simulink model "fig1"  (R2019b)
settings: Solver=VariableStepAuto  StartTime=0.0  StopTime=0.035  RelTol=1e-3
values from neighbouring files (symbols this model uses):
  f = 50    [Circuit_1.m]    (also in Circuit_2.m; Circuit_3_connected.m; Circuit_3_disconnected.m)
  V = (400*sqrt(2))/sqrt(3)    [Circuit_1.m]    (also in Circuit_2.m; Circuit_3_connected.m = (70*sqrt(2))/sqrt(3); Circuit_3_disconnected.m = (70*sqrt(2))/sqrt(3))
libraries: powerlib x8
settings Model: Creator=100448597  LastModifiedBy=robom
settings DataIOCC: SaveOutput=off  ReturnWorkspaceOutputs=off
settings SFSimCC: CustomCodeUndefinedFunction=UseInterfaceOnly

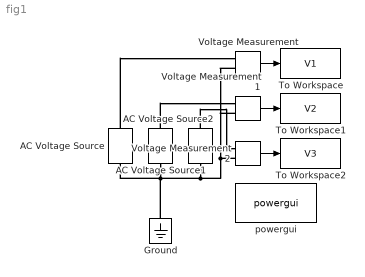
== system fig1 ==
  AC Voltage Source : powerlib/Electrical Sources/AC Voltage Source  Amplitude=V  Phase=0  Frequency=f  SampleTime=0  Measurements=None  BusType=swing  Pref=10e3  Qref=0  Qmin=-inf  Qmax=+inf
      settings: SourceProductName=Simscape Electrical
  AC Voltage Source1 : powerlib/Electrical Sources/AC Voltage Source  Amplitude=V  Phase=-120  Frequency=f  SampleTime=0  Measurements=None  BusType=swing  Pref=10e3  Qref=0  Qmin=-inf  Qmax=+inf
      settings: SourceProductName=Simscape Electrical
  AC Voltage Source2 : powerlib/Electrical Sources/AC Voltage Source  Amplitude=V  Phase=-240  Frequency=f  SampleTime=0  Measurements=None  BusType=swing  Pref=10e3  Qref=0  Qmin=-inf  Qmax=+inf
      settings: SourceProductName=Simscape Electrical
  Ground : powerlib/Elements/Ground  LConnTagsString=a
      settings: SourceProductName=Simscape Electrical
  To Workspace : ToWorkspace  VariableName=V1  SampleTime=-1
      settings: Save2DSignal=2-D array (concatenate along first dimension)
  To Workspace1 : ToWorkspace  VariableName=V2  SampleTime=-1
      settings: Save2DSignal=2-D array (concatenate along first dimension)
  To Workspace2 : ToWorkspace  VariableName=V3  SampleTime=-1
      settings: Save2DSignal=2-D array (concatenate along first dimension)
  Voltage Measurement : powerlib/Measurements/Voltage Measurement  PhasorSimulation=off  OutputType=Complex  PSBequivalent=0
      settings: SourceProductName=Simscape Electrical
  Voltage Measurement1 : powerlib/Measurements/Voltage Measurement  PhasorSimulation=off  OutputType=Complex  PSBequivalent=0
      settings: SourceProductName=Simscape Electrical
  Voltage Measurement2 : powerlib/Measurements/Voltage Measurement  PhasorSimulation=off  OutputType=Complex  PSBequivalent=0
      settings: SourceProductName=Simscape Electrical
  powergui : powerlib/powergui  Priority=1  SimulationMode=Continuous  SampleTime=50e-6  frequency=60  Iterations=50  frequencyindice=50  Pbase=100e6  ErrMax=1e-4  UnitsV=kV  UnitsW=MW  buscounter=0  FunctionMessages=off  echomessages=off  EnableUseOfTLC=off  CurrentSourceSwitches=off  DisableSnubberDevices=off  DisableRonSwitches=off  DisableVfSwitches=off  DisplayEquations=off  AutomaticDiscreteSolvers=off  SolverType=Tustin/Backward Euler (TBE)  Interpol=off  ExternalGateDelay=off  methode=off  Ts=100  x0status=blocks  SPID=on  SwTol=0  HookPort=off  NonlinearTolerance=0  nMaxIteration=15  ContinueOnMaxIteration=off  RestoreLinks=warning  ResistiveCurrentMeasurement=off  Frange=[0:2:500]  Ylog=off  Xlog=on  ShowGrid=off  save=off  variable=ZData  structure=0  ZoomFFT=off  StartTime=0.0  cycles=1  DisplayStyle=1  fundamental=60  FreqAxis=off  MaxFrequency=1000  frequencyindicesteady=1  RmsSteady=1  display=off
      settings: SourceProductName=Simscape Electrical
  wires:
  Voltage Measurement/1 -> To Workspace/1
  Voltage Measurement1/1 -> To Workspace1/1
  Voltage Measurement2/1 -> To Workspace2/1
  connections:
  AC Voltage Source1/LConn1 -- Ground/LConn1 -- Voltage Measurement/LConn2 -- Voltage Measurement1/LConn2 -- Voltage Measurement2/LConn2 -- AC Voltage Source2/LConn1 -- AC Voltage Source/LConn1
  AC Voltage Source/RConn1 -- Voltage Measurement/LConn1
  AC Voltage Source1/RConn1 -- Voltage Measurement1/LConn1
  AC Voltage Source2/RConn1 -- Voltage Measurement2/LConn1
